simulink model "UAV_log"  (R2019b)
settings: Solver=FixedStepAuto  StartTime=0.0  StopTime=100  RelTol=1e-3
InitFcn:
  | load('BusDefinitions.mat')
values from neighbouring files (symbols this model uses):
  q_single = cov(out.In_Out_Data{1}.Values.Data)    [calculate_controller_gain.m]
  r_single = cov(out.In_Out_Data{2}.Values.Data)    [calculate_controller_gain.m]
undefined symbols (not defined in the file or in its folder): A_s_double, A_s_single, B_s_double, B_s_single, C_double, C_single, codertarget, D_double, D_single, Discrete, omega_c, Time, Ts
libraries: ctrlSharedLib x5
settings Model: ExtModeTrigDuration=80  Creator=Sankalp Bhan  LastModifiedBy=Chris
settings OptimizationCC: PassReuseOutputArgsThreshold=0  MaxStackSize=64
settings DebuggingCC: ParameterTunabilityLossMsg=error  ArithmeticOperatorsInVariantConditions=warning
settings HardwareCC: ProdBitPerPointer=32  ProdBitPerSizeT=32  ProdBitPerPtrDiffT=32  ProdLargestAtomicInteger=Long  ProdWordSize=32  ProdHWDeviceType=ARM Compatible->ARM 9  UseEmbeddedCoderFeatures=off
settings SFSimCC: SimUseLocalCustomCode=off  MATLABDynamicMemAlloc=off
settings RTWCC: SystemTargetFile=ert.tlc  HardwareBoard=PARROT Mambo  TLCOptions="-aInlineSetEventsForThisBaseRateFcn=TLC_FALSE -aSuppressMultiTaskScheduler=TLC_FALSE   -aRateBasedStepFcn=1"  TemplateMakefile=ert_default_tmf  GenerateReport=on  RTWUseLocalCustomCode=off  Toolchain=Sourcery G++ Lite GNU Toolchain for Drones  LaunchReport=on
settings CodeAppCC: ForceParamTrailComments=on  OperatorAnnotations=on  StateflowObjectComments=on
settings ERTTargetCC: ERTCustomFileBanners=off  MatFileLogging=on  SupportContinuousTime=on  SupportNonInlinedSFcns=on  RemoveResetFunc=off  ModelStepFunctionPrototypeControlCompliant=off

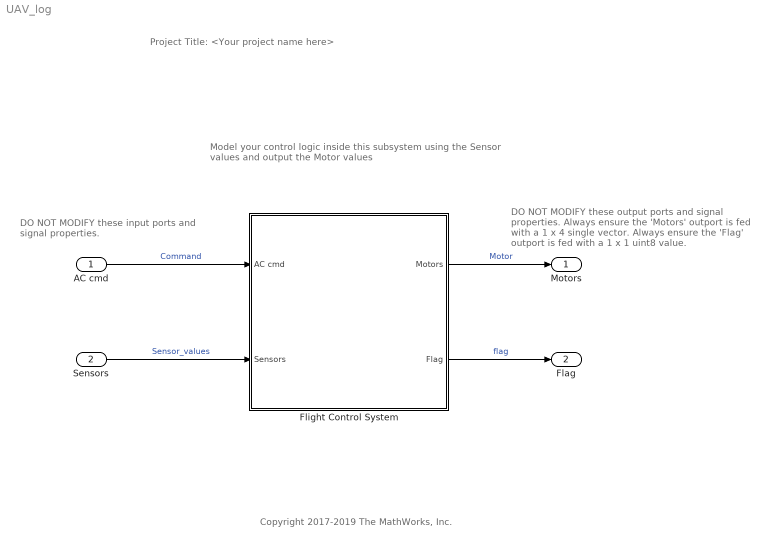
== system UAV_log ==
  note: Model your control logic inside this subsystem
      | using the Sensor values and output the
      | Motor values
  note: DO NOT MODIFY these output ports
      | and signal properties.
      |
      |
      |
      | Always ensure the 'Motors' outport
      | is fed with a 1 x 4 single vector.
      |
      |
      |
      |
      |
      | Always ensure the 'Flag' outport is
      | fed with a 1 x 1 uint8 value.
  note: DO NOT MODIFY these input
      | ports and signal properties.
  note: Copyright 2017-2019 The MathWorks, Inc.
  note: Project Title: <Your project name here>
  AC cmd : Inport  OutDataTypeStr=Bus: CommandBus  BusOutputAsStruct=on
  Sensors : Inport  Port=2  OutDataTypeStr=Bus: SensorsBus  BusOutputAsStruct=on
  Flight Control System : Subsystem  InitFcn=codertarget.parrot.internal.fcsSubsystemCallback(gcb);
  Motors : Outport  OutDataTypeStr=single  PortDimensions=[1 4]  VectorParamsAs1DForOutWhenUnconnected=off
  Flag : Outport  Port=2  OutDataTypeStr=uint8  PortDimensions=1  VectorParamsAs1DForOutWhenUnconnected=off
  wires:
  Flight Control System/1(Motors) -> Motors/1  "Motor"
  AC cmd/1 -> Flight Control System/1(AC cmd)  "Command"
  Sensors/1 -> Flight Control System/2(Sensors)  "Sensor_values"
  Flight Control System/2(Flag) -> Flag/1  "flag"

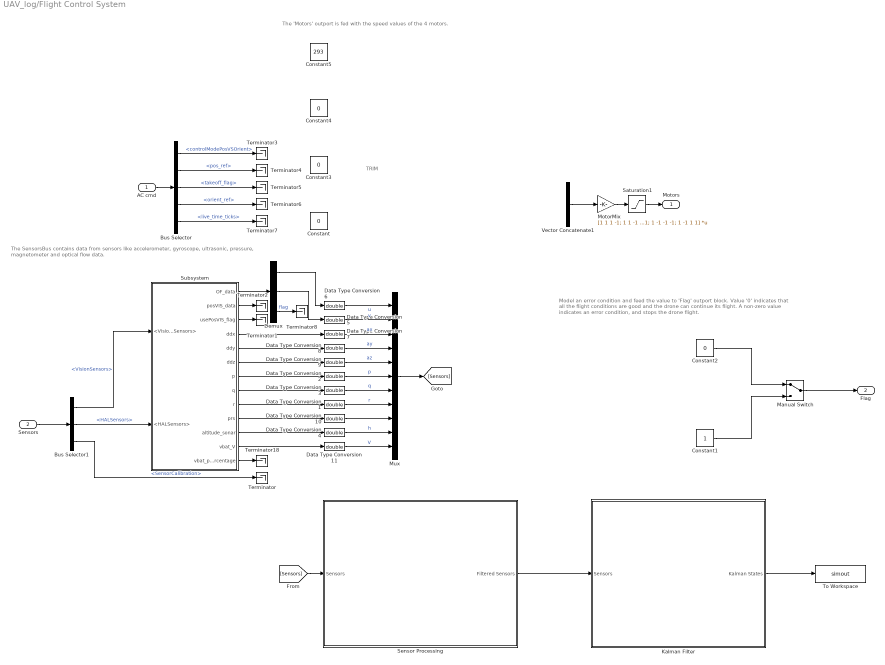
== system UAV_log/Flight Control System ==
  note: TRIM
  note: The 'Motors' outport is fed with the speed values of the 4 motors.
  note: Model an error condition and feed the value to 'Flag' outport block.
      | Value '0' indicates that all the flight conditions are good and the drone
      | can continue its flight.
      | A non-zero value indicates an error condition, and stops the drone
      | flight.
  note: The SensorsBus contains data from sensors like
      | accelerometer, gyroscope, ultrasonic, pressure,
      | magnetometer and optical flow data.
  AC cmd : Inport
  Sensors : Inport  Port=2
  Bus Selector : BusSelector  OutputSignals=controlModePosVSOrient,pos_ref,takeoff_flag,orient_ref,live_time_ticks
  Bus Selector1 : BusSelector  OutputSignals=VisionSensors,HALSensors,SensorCalibration
  Constant : Constant  Value=0  SampleTime=Ts
  Constant1 : Constant  OutDataTypeStr=uint8
  Constant2 : Constant  Value=0  OutDataTypeStr=uint8
  Constant3 : Constant  Value=0  SampleTime=Ts
  Constant4 : Constant  Value=0  SampleTime=Ts
  Constant5 : Constant  Value=293  SampleTime=Ts
  Data Type Conversion{1..11} (11 alike) : DataTypeConversion  OutDataTypeStr=double
  Demux : Demux  Outputs=3
  Kalman Filter : Subsystem
  Manual Switch : ManualSwitch
  MotorMix : Gain  Gain=[1 1 1 -1; 1 1 -1 1; 1 -1 -1 -1; 1 -1 1 1]  Multiplication=Matrix(K*u)
  Mux : Mux  Inputs=11
  Saturation1 : Saturate  UpperLimit=500  LowerLimit=0  OutDataTypeStr=single
  "Sensor Processing " : Subsystem
  Subsystem : Subsystem
  Terminator{,1..8,18} (10 alike) : Terminator
  To Workspace : ToWorkspace  VariableName=simout  SaveFormat=Structure With Time  SampleTime=-1
  Vector Concatenate1 : Concatenate  NumInputs=4
  Motors : Outport  VectorParamsAs1DForOutWhenUnconnected=off
  Flag : Outport  Port=2  VectorParamsAs1DForOutWhenUnconnected=off
  wires:
  AC cmd/1 -> Bus Selector/1
  Sensors/1 -> Bus Selector1/1
  Bus Selector/1 -> Terminator3/1  "<controlModePosVSOrient>"
  Bus Selector/2 -> Terminator4/1  "<pos_ref>"
  Bus Selector/3 -> Terminator5/1  "<takeoff_flag>"
  Bus Selector/4 -> Terminator6/1  "<orient_ref>"
  Bus Selector/5 -> Terminator7/1  "<live_time_ticks>"
  Manual Switch/1 -> Flag/1
  Constant2/1 -> Manual Switch/1
  Constant1/1 -> Manual Switch/2
  Vector Concatenate1/1 -> MotorMix/1
  Saturation1/1 -> Motors/1
  Bus Selector1/1 -> Subsystem/1(<VisionSensors>)  "<VisionSensors>"
  Bus Selector1/2 -> Subsystem/2(<HALSensors>)  "<HALSensors>"
  Bus Selector1/3 -> Terminator/1  "<SensorCalibration>"
  Subsystem/1(OF_data) -> Demux/1
  Subsystem/4(ddx) -> Data Type Conversion7/1
  Subsystem/5(ddy) -> Data Type Conversion8/1
  Subsystem/6(ddz) -> Data Type Conversion9/1
  Subsystem/7(p) -> Data Type Conversion2/1
  Subsystem/9(r) -> Data Type Conversion1/1
  Subsystem/11(altitude_sonar) -> Data Type Conversion4/1
  Subsystem/12(vbat_V) -> Data Type Conversion11/1
  Subsystem/13(vbat_percentage) -> Terminator18/1
  Subsystem/8(q) -> Data Type Conversion3/1
  Mux/1 -> [Sensors]
  MotorMix/1 -> Saturation1/1
  Subsystem/3(usePosVIS_flag) -> Terminator1/1
  Subsystem/2(posVIS_data) -> Terminator2/1
  Demux/1 -> Data Type Conversion6/1
  Demux/2 -> Data Type Conversion5/1
  Demux/3 -> Terminator8/1  "flag"
  Subsystem/10(prs) -> Data Type Conversion10/1
  Data Type Conversion1/1 -> Mux/8  "r"
  Data Type Conversion2/1 -> Mux/6  "p"
  Data Type Conversion3/1 -> Mux/7  "q"
  Data Type Conversion4/1 -> Mux/10  "h"
  Data Type Conversion5/1 -> Mux/2  "v"
  Data Type Conversion6/1 -> Mux/1  "u"
  Data Type Conversion7/1 -> Mux/3  "ax"
  Data Type Conversion8/1 -> Mux/4  "ay"
  Data Type Conversion9/1 -> Mux/5  "az"
  Data Type Conversion10/1 -> Mux/9
  Data Type Conversion11/1 -> Mux/11  "V"
  [Sensors] -> "Sensor Processing "/1(Sensors)
  "Sensor Processing "/1(Filtered Sensors) -> Kalman Filter/1(Sensors)
  Kalman Filter/1(Kalman States) -> To Workspace/1

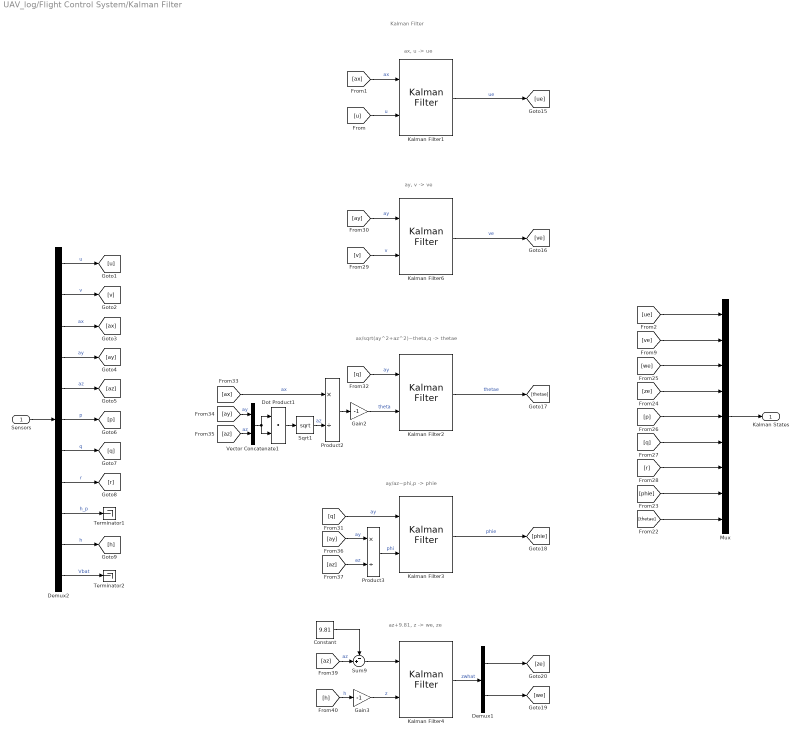
== system UAV_log/Flight Control System/Kalman Filter ==
  note: ay/az~phi,p -> phie
  note: ax/sqrt(ay^2+az^2)~theta,q -> thetae
  note: ax, u -> ue
  note: az+9.81, z -> we, ze
  note: ay, v -> ve
  note: Kalman Filter
  Sensors : Inport
  Constant : Constant  Value=9.81  SampleTime=0.005
  Demux1 : Demux  Outputs=2
  Demux2 : Demux  Outputs=11
  Dot Product1 : DotProduct  OutMin=0.0001  InputSameDT=on  OutDataTypeStr=Inherit: Inherit via internal rule
  Gain2 : Gain  Gain=-1
  Gain3 : Gain  Gain=-1
  Kalman Filter{1..3,6} (4 alike) : ctrlSharedLib/Kalman Filter  TimeDomain=Discrete-Time  UseCurrentEstimator=on  ModelSource=Individual A, B, C, D matrices  ModelSourceVariable=ss(0.95,1,1,0,1)  A=A_s_single  B=B_s_single  C=C_single  D=D_single  NumberOfStates=1  NumberOfInputs=1  NumberOfOutputs=1  InitialEstimateSource=Dialog  X0=[0]  P0=10  UseK=off  UseGH=off  NumberOfProcessNoiseInputs=1  G=1  TimeInvariantG=on  H=0  TimeInvariantH=on  Q=[1]*q_single  TimeInvariantQ=on  R=[1]*r_single*10000  TimeInvariantR=on  N=0  TimeInvariantN=on  AddInputPort=on  AddEnablePort=off  OutputEstimatedY=off  OutputP=off  Ts=Ts
      settings: SourceProductBaseCode=CT
  Kalman Filter4 : ctrlSharedLib/Kalman Filter  TimeDomain=Discrete-Time  UseCurrentEstimator=on  ModelSource=Individual A, B, C, D matrices  ModelSourceVariable=ss(0.95,1,1,0,1)  A=A_s_double  B=B_s_double  C=C_double  D=D_double  NumberOfStates=1  NumberOfInputs=1  NumberOfOutputs=1  InitialEstimateSource=Dialog  X0=[0]  P0=10  UseK=off  UseGH=off  NumberOfProcessNoiseInputs=1  G=1  TimeInvariantG=on  H=0  TimeInvariantH=on  Q=[0 0; 0 1]*q_single  TimeInvariantQ=on  R=[1]*r_single*10000  TimeInvariantR=on  N=0  TimeInvariantN=on  AddInputPort=on  AddEnablePort=off  OutputEstimatedY=off  OutputP=off  Ts=Ts
      settings: SourceProductBaseCode=CT
  Mux : Mux  Inputs=9
  Product2 : Product  Inputs=*/
  Product3 : Product  Inputs=*/
  Sqrt1 : Sqrt  SaturateOnIntegerOverflow=on
  Sum9 : Sum  Inputs=-+|
  Terminator1 : Terminator
  Terminator2 : Terminator
  Vector Concatenate1 : Concatenate
  Kalman States : Outport
  wires:
  Demux2/9 -> Terminator1/1  "h_p"
  Demux2/1 -> [u]  "u"
  Demux2/4 -> [ay]  "ay"
  Demux2/3 -> [ax]  "ax"
  Sensors/1 -> Demux2/1
  Demux2/2 -> [v]  "v"
  Demux2/10 -> [h]  "h"
  Demux2/5 -> [az]  "az"
  Demux2/7 -> [q]  "q"
  Demux2/8 -> [r]  "r"
  Demux2/6 -> [p]  "p"
  Demux2/11 -> Terminator2/1  "Vbat"
  [ue] -> Mux/1
  [ve] -> Mux/2
  [we] -> Mux/3
  [ze] -> Mux/4
  Mux/1 -> Kalman States/1
  [r] -> Mux/7
  [q] -> Mux/6
  [p] -> Mux/5
  [phie] -> Mux/8
  [thetae] -> Mux/9
  Sqrt1/1 -> Product2/2  "az"
  Gain3/1 -> Kalman Filter4/2  "z"
  Kalman Filter4/1 -> Demux1/1  "zwhat"
  [ax] -> Product2/1  "ax"
  [v] -> Kalman Filter6/2  "v"
  Kalman Filter2/1 -> [thetae]  "thetae"
  [u] -> Kalman Filter1/2  "u"
  [ay] -> Kalman Filter6/1  "ay"
  Gain2/1 -> Kalman Filter2/2  "theta"
  [ay] -> Product3/1  "ay"
  Dot Product1/1 -> Sqrt1/1
  Product2/1 -> Gain2/1
  Demux1/2 -> [we]
  [ay] -> Vector Concatenate1/1  "ay"
  [az] -> Vector Concatenate1/2  "az"
  Vector Concatenate1/1 -> Dot Product1/1, Dot Product1/2
  Product3/1 -> Kalman Filter3/2  "phi"
  Demux1/1 -> [ze]
  Kalman Filter6/1 -> [ve]  "ve"
  [h] -> Gain3/1  "h"
  [q] -> Kalman Filter3/1  "ay"
  Kalman Filter1/1 -> [ue]  "ue"
  [q] -> Kalman Filter2/1  "ay"
  Kalman Filter3/1 -> [phie]  "phie"
  [az] -> Product3/2  "az"
  Sum9/1 -> Kalman Filter4/1
  Constant/1 -> Sum9/1
  [az] -> Sum9/2  "az"
  [ax] -> Kalman Filter1/1  "ax"

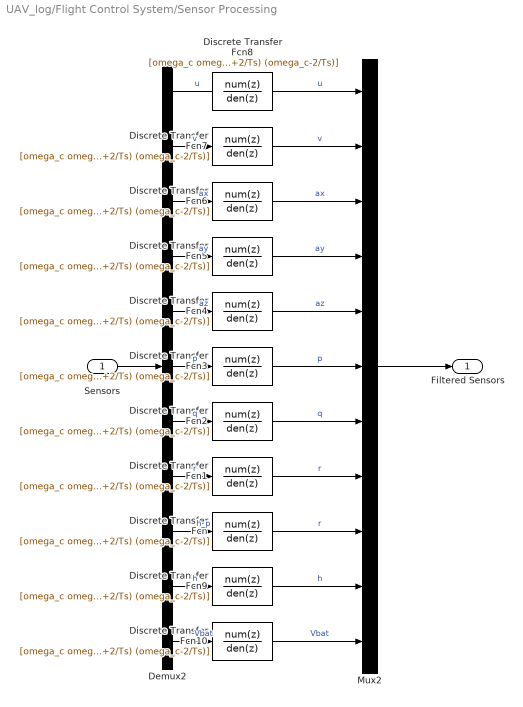
== system UAV_log/Flight Control System/Sensor Processing  ==
  Sensors : Inport
  Demux2 : Demux  Outputs=11
  Discrete Transfer Fcn{,1..10} (11 alike) : DiscreteTransferFcn  Numerator=[omega_c omega_c]  Denominator=[(omega_c+2/Ts) (omega_c-2/Ts)]  SampleTime=0.005
  Mux2 : Mux  Inputs=11
  Filtered Sensors : Outport
  wires:
  Mux2/1 -> Filtered Sensors/1
  Demux2/2 -> Discrete Transfer Fcn7/1  "v"
  Discrete Transfer Fcn9/1 -> Mux2/10  "h"
  Demux2/11 -> Discrete Transfer Fcn10/1  "Vbat"
  Sensors/1 -> Demux2/1
  Demux2/6 -> Discrete Transfer Fcn3/1  "p"
  Discrete Transfer Fcn2/1 -> Mux2/7  "q"
  Demux2/3 -> Discrete Transfer Fcn6/1  "ax"
  Demux2/4 -> Discrete Transfer Fcn5/1  "ay"
  Demux2/1 -> ?  "u"
  Discrete Transfer Fcn7/1 -> Mux2/2  "v"
  Demux2/8 -> Discrete Transfer Fcn1/1  "r"
  Discrete Transfer Fcn8/1 -> Mux2/1  "u"
  Discrete Transfer Fcn5/1 -> Mux2/4  "ay"
  Discrete Transfer Fcn1/1 -> Mux2/8  "r"
  Demux2/10 -> Discrete Transfer Fcn9/1  "h"
  Discrete Transfer Fcn4/1 -> Mux2/5  "az"
  Demux2/7 -> Discrete Transfer Fcn2/1  "q"
  Discrete Transfer Fcn10/1 -> Mux2/11  "Vbat"
  Discrete Transfer Fcn3/1 -> Mux2/6  "p"
  Demux2/5 -> Discrete Transfer Fcn4/1  "az"
  Discrete Transfer Fcn6/1 -> Mux2/3  "ax"
  Demux2/9 -> Discrete Transfer Fcn/1  "h_p"
  Discrete Transfer Fcn/1 -> Mux2/9  "r"

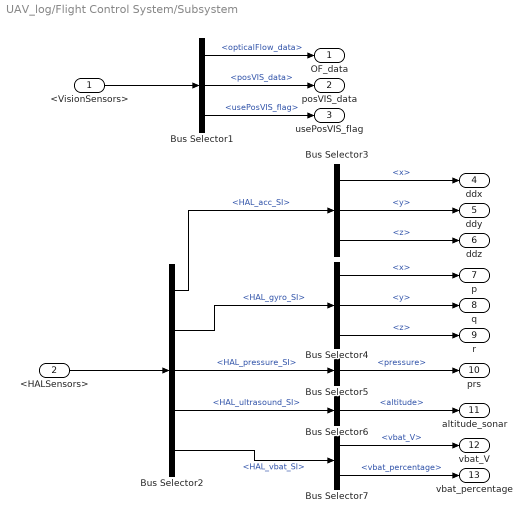
== system UAV_log/Flight Control System/Subsystem ==
  <VisionSensors> : Inport
  <HALSensors> : Inport  Port=2
  Bus Selector1 : BusSelector  OutputSignals=opticalFlow_data,posVIS_data,usePosVIS_flag
  Bus Selector2 : BusSelector  OutputSignals=HAL_acc_SI,HAL_gyro_SI,HAL_pressure_SI,HAL_ultrasound_SI,HAL_vbat_SI
  Bus Selector3 : BusSelector  OutputSignals=x,y,z
  Bus Selector4 : BusSelector  OutputSignals=x,y,z
  Bus Selector5 : BusSelector  OutputSignals=pressure
  Bus Selector6 : BusSelector  OutputSignals=altitude
  Bus Selector7 : BusSelector  OutputSignals=vbat_V,vbat_percentage
  OF_data : Outport  VectorParamsAs1DForOutWhenUnconnected=off
  posVIS_data : Outport  Port=2  VectorParamsAs1DForOutWhenUnconnected=off
  usePosVIS_flag : Outport  Port=3  VectorParamsAs1DForOutWhenUnconnected=off
  ddx : Outport  Port=4  VectorParamsAs1DForOutWhenUnconnected=off
  ddy : Outport  Port=5  VectorParamsAs1DForOutWhenUnconnected=off
  ddz : Outport  Port=6  VectorParamsAs1DForOutWhenUnconnected=off
  p : Outport  Port=7  VectorParamsAs1DForOutWhenUnconnected=off
  q : Outport  Port=8  VectorParamsAs1DForOutWhenUnconnected=off
  r : Outport  Port=9  VectorParamsAs1DForOutWhenUnconnected=off
  prs : Outport  Port=10  VectorParamsAs1DForOutWhenUnconnected=off
  altitude_sonar : Outport  Port=11  VectorParamsAs1DForOutWhenUnconnected=off
  vbat_V : Outport  Port=12  VectorParamsAs1DForOutWhenUnconnected=off
  vbat_percentage : Outport  Port=13  VectorParamsAs1DForOutWhenUnconnected=off
  wires:
  <VisionSensors>/1 -> Bus Selector1/1
  <HALSensors>/1 -> Bus Selector2/1
  Bus Selector1/1 -> OF_data/1  "<opticalFlow_data>"
  Bus Selector1/2 -> posVIS_data/1  "<posVIS_data>"
  Bus Selector1/3 -> usePosVIS_flag/1  "<usePosVIS_flag>"
  Bus Selector2/1 -> Bus Selector3/1  "<HAL_acc_SI>"
  Bus Selector2/2 -> Bus Selector4/1  "<HAL_gyro_SI>"
  Bus Selector2/3 -> Bus Selector5/1  "<HAL_pressure_SI>"
  Bus Selector2/4 -> Bus Selector6/1  "<HAL_ultrasound_SI>"
  Bus Selector2/5 -> Bus Selector7/1  "<HAL_vbat_SI>"
  Bus Selector3/1 -> ddx/1  "<x>"
  Bus Selector3/2 -> ddy/1  "<y>"
  Bus Selector3/3 -> ddz/1  "<z>"
  Bus Selector4/2 -> q/1  "<y>"
  Bus Selector4/1 -> p/1  "<x>"
  Bus Selector4/3 -> r/1  "<z>"
  Bus Selector5/1 -> prs/1  "<pressure>"
  Bus Selector6/1 -> altitude_sonar/1  "<altitude>"
  Bus Selector7/1 -> vbat_V/1  "<vbat_V>"
  Bus Selector7/2 -> vbat_percentage/1  "<vbat_percentage>"
